simulink model "Week09-lqr_simulink"  (R2022a)
settings: Solver=VariableStepAuto  StartTime=0.0  StopTime=5.0  RelTol=1e-3
settings Model: Creator=Kim  LastModifiedBy=Kim

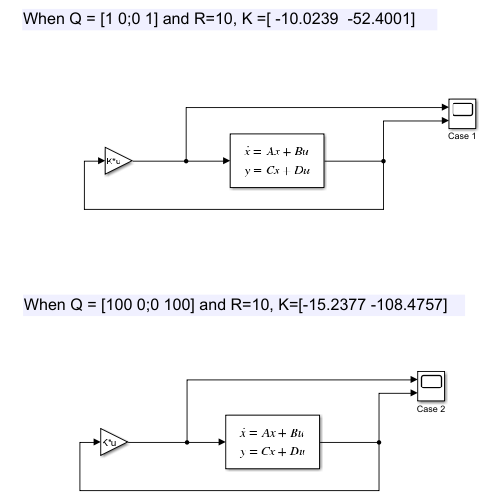
[thumbnail: Simulink's stored preview of the top-level diagram]
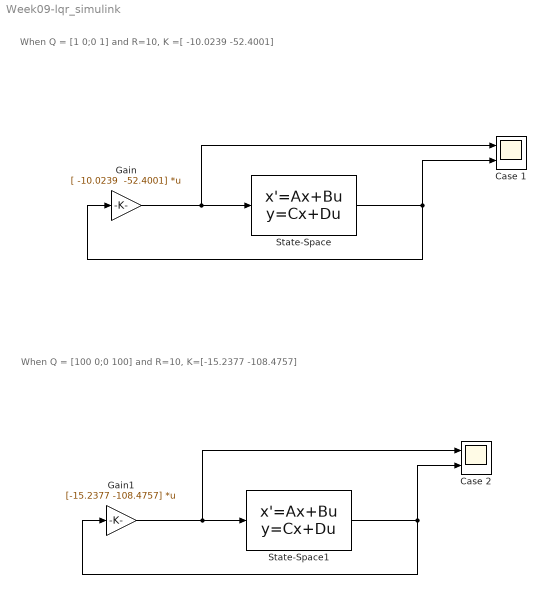
== system Week09-lqr_simulink ==
  note: When Q = [1 0;0 1] and R=10, K =[ -10.0239 -52.4001]
  note: When Q = [100 0;0 100] and R=10, K=[-15.2377 -108.4757]
  Case 1 : Scope  NumInputPorts=2
  Case 2 : Scope  NumInputPorts=2
  Gain : Gain  Gain="[ -10.0239  -52.4001]"  Multiplication=Matrix(K*u)
  Gain1 : Gain  Gain=[-15.2377 -108.4757]  Multiplication=Matrix(K*u)
  State-Space : StateSpace  A=[1, -2;1, 4]  B=[1; 0.1]  C=[1, 0;0, 1]  D=[0;0]  InitialCondition=[1; -1]
  State-Space1 : StateSpace  A=[1, -2;1, 4]  B=[1; 0.1]  C=[1, 0;0, 1]  D=[0;0]  InitialCondition=[1; -1]
  wires:
  Gain/1 -> Case 1/1, State-Space/1
  State-Space/1 -> Case 1/2, Gain/1
  State-Space1/1 -> Case 2/2, Gain1/1
  Gain1/1 -> Case 2/1, State-Space1/1
